simulink model "ForkMemory3Edges323"  (Simulink 7.6)
settings: Solver=ode45  StartTime=0.0  StopTime=10.0  RelTol=1e-3
settings Model: Creator=DominikC  LastModifiedBy=DominikC

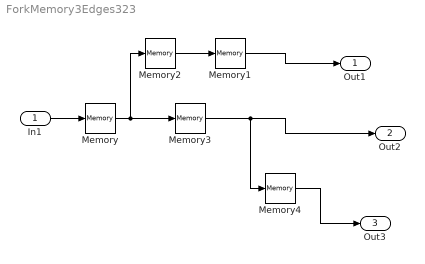
== system ForkMemory3Edges323 ==
  In1 : Inport
  Memory{,1..4} (5 alike) : Memory
  Out1 : Outport
  Out2 : Outport  Port=2
  Out3 : Outport  Port=3
  wires:
  In1/1 -> Memory/1
  Memory/1 -> Memory3/1, Memory2/1
  Memory2/1 -> Memory1/1
  Memory3/1 -> Out2/1, Memory4/1
  Memory1/1 -> Out1/1
  Memory4/1 -> Out3/1
